simulink model "closed_loop_diagram_2"  (R2023b)
settings: Solver=VariableStepAuto  StartTime=0.0  StopTime=80  RelTol=1e-3
values from neighbouring files (symbols this model uses):
  A = [0   1 ... (first row only)    [DC_motor_example_LQR_v2.m]    (also in inverted_pendulum_main.m = [ 0         0               1                   0)
  B = [0 ... (first row only)    [DC_motor_example_LQR_v2.m]    (also in inverted_pendulum_main.m = [       0)
  Cc = eye(4)    [inverted_pendulum_main.m]
  Dc = zeros(4, 1)    [inverted_pendulum_main.m]
  K = lqr(A,B,Q,R)    [DC_motor_example_LQR_v2.m]    (also in inverted_pendulum_main.m = lqr(sys, Qf, Rf))
  Ts = 0.005    [inverted_pendulum_main.m]
  wc = pi    (= 3.14159265359)    [inverted_pendulum_main.m]
undefined symbols (not defined in the file or in its folder): x_desired
libraries: simulink x2
settings Model: Creator=loicdewit  LastModifiedBy=loicdewit

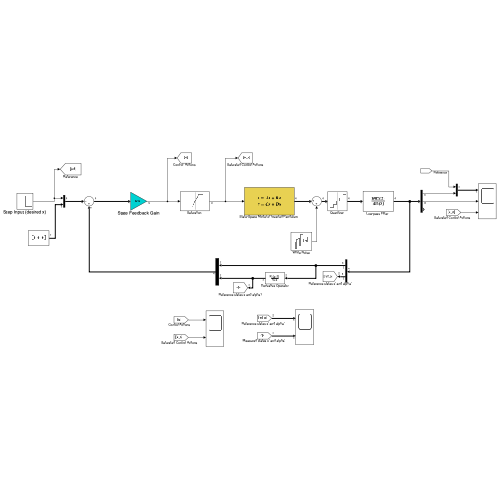
[thumbnail: Simulink's stored preview of the top-level diagram]
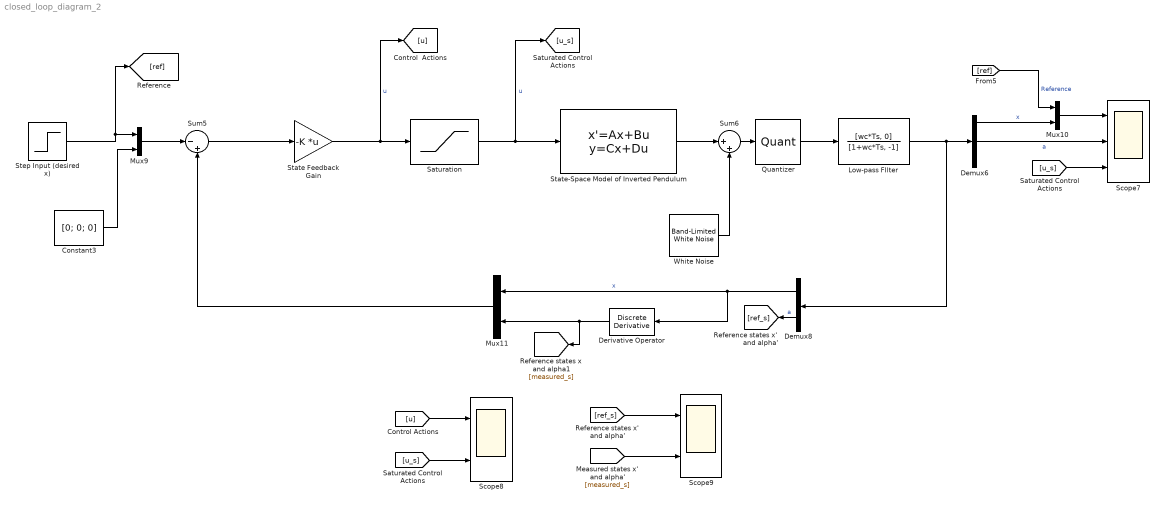
== system closed_loop_diagram_2 ==
  Constant3 : Constant  Value=[0; 0; 0]  SampleTime=Ts
  Demux6 : Demux  Outputs=[1 1 2]
  Demux8 : Demux  Outputs="[2  -1]"
  Derivative Operator : simulink/Discrete/Discrete Derivative  gainval=1.0  ICPrevScaledInput=0.0  OutMin=[]  OutMax=[]  OutDataType=fixdt(1, 16)  OutScaling=2^-10  DoSatur=off
  "Low-pass FIlter  " : DiscreteTransferFcn  Numerator=[wc*Ts, 0]  Denominator=[1+wc*Ts, -1]
  Mux10 : Mux  Inputs=2
  Mux11 : Mux  Inputs=2
  Mux9 : Mux  Inputs=2
  "Quantizer " : Quantizer  QuantizationInterval=20/(2^16)
  "Saturation " : Saturate  UpperLimit=5  LowerLimit=-5
  Scope7 : Scope  NumInputPorts=3
  Scope8 : Scope  NumInputPorts=2
  Scope9 : Scope  NumInputPorts=2
  State Feedback Gain : Gain  Gain=-K  Multiplication=Matrix(K*u)
  "State-Space Model of Inverted Pendulum " : StateSpace  A=A  B=B  C=Cc  D=Dc  InitialCondition=0
  Step Input (desired x) : Step  Time=20  After=x_desired  SampleTime=Ts
  Sum5 : Sum  Inputs=|-+
  Sum6 : Sum  Inputs=|++
  White Noise : simulink/Sources/Band-Limited White Noise  Cov=[0.00001 * Ts]  Ts=Ts  seed=[13072002]  VectorParams1D=off
  wires:
  Demux6/2 -> Scope7/2  "a"
  Mux9/1 -> Sum5/1
  Constant3/1 -> Mux9/2
  Step Input (desired x)/1 -> [ref], Mux9/1
  [u_s] -> Scope7/3
  Sum5/1 -> State Feedback Gain/1
  Mux10/1 -> Scope7/1
  Demux6/1 -> Mux10/2  "x"
  [ref] -> Mux10/1  "Reference"
  Sum6/1 -> "Quantizer "/1
  Mux11/1 -> Sum5/2
  State Feedback Gain/1 -> [u], "Saturation "/1  "u"
  "Saturation "/1 -> [u_s], "State-Space Model of Inverted Pendulum "/1  "u"
  White Noise/1 -> Sum6/2
  "Quantizer "/1 -> "Low-pass FIlter  "/1
  "Low-pass FIlter  "/1 -> Demux8/1, Demux6/1
  "State-Space Model of Inverted Pendulum "/1 -> Sum6/1
  Derivative Operator/1 -> Mux11/2, [measured_s]
  Demux8/1 -> Derivative Operator/1, Mux11/1  "x"
  [u] -> Scope8/1
  [u_s] -> Scope8/2
  Demux8/2 -> [ref_s]  "a"
  [ref_s] -> Scope9/1
  [measured_s] -> Scope9/2
